simulink model "joystick_test"  (R2021a)
settings: Solver=VariableStepAuto  StartTime=0.0  StopTime=inf  RelTol=1e-3
libraries: vrlib x2
settings Model: Creator=ozuem  LastModifiedBy=ozuem

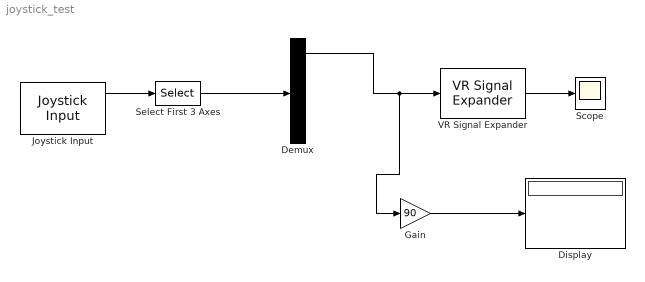
== system joystick_test ==
  Demux : Demux  Outputs=6
  Display : Display
  Gain : Gain  Gain=90
  Joystick Input : vrlib/Joystick Input  joyid=1  adjustports=on  forcefeed=off
  Scope : Scope
  Select First 3 Axes : Selector  InputPortWidth=6  IndexOptions=Index vector (dialog)  Indices=[1 2 3 4 5 6]  OutputSizes=1
      settings: AttributesFormatString=(Joystick - dependent)
  VR Signal Expander : vrlib/VR Signal Expander  outwidth=4  outidx=[2 4]
  wires:
  Joystick Input/1 -> Select First 3 Axes/1
  Select First 3 Axes/1 -> Demux/1
  VR Signal Expander/1 -> Scope/1
  Gain/1 -> Display/1
  Demux/1 -> Gain/1, VR Signal Expander/1
